simulink model "SunSensor"  (R2025b)
settings: Solver=VariableStepAuto  StartTime=0.0  StopTime=10  RelTol=1e-3
settings Model: Creator=brien  LastModifiedBy=chass

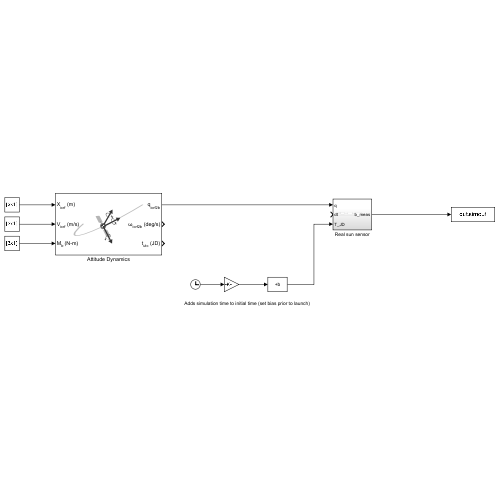
[thumbnail: Simulink's stored preview of the top-level diagram]
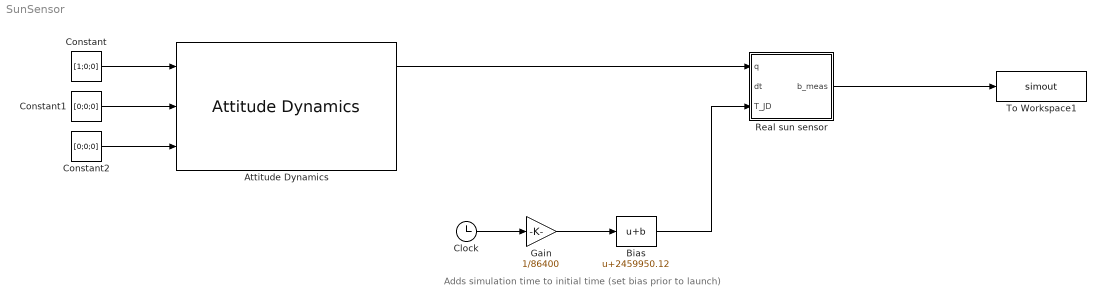
== system SunSensor ==
  note: Adds simulation time to initial time (set bias prior to launch)
  Attitude Dynamics : AttitudeDynamics
  Bias : Bias  Bias=2459950.12  SaturateOnIntegerOverflow=off
  Clock : Clock
  Constant : Constant  Value=[1;0;0]  VectorParams1D=off
  Constant1 : Constant  Value=[0;0;0]  VectorParams1D=off
  Constant2 : Constant  Value=[0;0;0]  VectorParams1D=off
  Gain : Gain  Gain=1/86400
  Real sun sensor : Subsystem
  To Workspace1 : ToWorkspace  VariableName=simout  SampleTime=-1
  wires:
  Constant/1 -> Attitude Dynamics/1
  Constant1/1 -> Attitude Dynamics/2
  Constant2/1 -> Attitude Dynamics/3
  Clock/1 -> Gain/1
  Gain/1 -> Bias/1
  Attitude Dynamics/1 -> Real sun sensor/1(q)
  Bias/1 -> Real sun sensor/3(T_JD)
  Real sun sensor/1(b_meas) -> To Workspace1/1

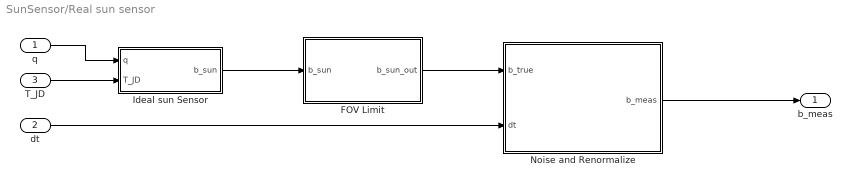
== system SunSensor/Real sun sensor ==
  q : Inport
  dt : Inport  Port=2
  T_JD : Inport  Port=3
  FOV Limit : MATLAB Function  TreatAsAtomicUnit=on
  Ideal sun Sensor : Subsystem
  Noise and Renormalize : MATLAB Function  TreatAsAtomicUnit=on
  b_meas : Outport
  wires:
  dt/1 -> Noise and Renormalize/2(dt)
  Ideal sun Sensor/1(b_sun) -> FOV Limit/1(b_sun)
  FOV Limit/1(b_sun_out) -> Noise and Renormalize/1(b_true)
  Noise and Renormalize/1(b_meas) -> b_meas/1
  T_JD/1 -> Ideal sun Sensor/2(T_JD)
  q/1 -> Ideal sun Sensor/1(q)

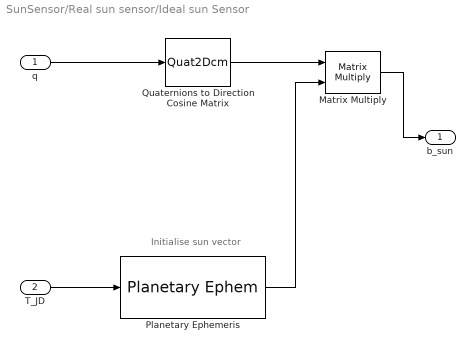
== system SunSensor/Real sun sensor/Ideal sun Sensor ==
  note: Initialise sun vector
  q : Inport
  T_JD : Inport  Port=2
  Matrix Multiply : Product  Multiplication=Matrix(*)
  Planetary Ephemeris : PlanetaryEphem  units=m,m/s  target=Sun  outputVelocity=off
  Quaternions to Direction Cosine Matrix : Quat2Dcm
  b_sun : Outport
  wires:
  q/1 -> Quaternions to Direction Cosine Matrix/1
  Quaternions to Direction Cosine Matrix/1 -> Matrix Multiply/1
  Matrix Multiply/1 -> b_sun/1
  Planetary Ephemeris/1 -> Matrix Multiply/2
  T_JD/1 -> Planetary Ephemeris/1

== matlab function SunSensor/Real sun sensor/Noise and Renormalize ==
  settings: updateMethod=DISCRETE
  data: b_true input; b_meas output; dt input
function b_meas = sunSensorVector(b_true, dt)
% b_true : 3x1 true Sun vector (unit vector) in the body frame of reference ?
% dt     : simulation timestep (s)

% Output:
% b_meas : 3x1 measured Sun vector (unit vector) in the body frame of reference ?
%          with noise, slew-rate limit, and normalized

    sigma_angle = deg2rad(0.1);   % 1-sigma noise (from 0.2° 2-sigma spec)
    slew_max    = deg2rad(70);    % max change per second

    
    % 1) Add Gaussian noise (small vector perturbation)
    
    noise = sigma_angle * randn(3,1);
    b_noisy = b_true(:) + noise;

    
    % 2) Apply slew-rate limit
    
    persistent b_prev;
    if isempty(b_prev)
        b_prev = b_noisy;
    end

    delta = b_noisy - b_prev;
    delta_norm = norm(delta);
    max_step = slew_max * dt;

    if delta_norm > max_step
        delta = delta * (max_step / delta_norm);
    end

    b_slew = b_prev + delta;
    b_prev = b_slew;

    
    % 3) Normalize to unit vector
    
    b_meas = b_slew / norm(b_slew);

end

== matlab function SunSensor/Real sun sensor/FOV Limit ==
  data: b_sun input; b_sun_out output
function b_sun_out = sunSensorFOV(b_sun)
    % Sun Sensor FOV Implementation
    %
    % Input:
    %   b_sun       - 3x1 Sun vector in body frame
    % Output:
    %   b_sun_out   - 3x1 Sun vector with FOV applied

    % --- Parameters ---
    alpha = 180;                 % FOV half-angle in degrees
    sensor_axis = [1; 0; 0];    % Sensor pointing along body x-axis

    % Normalize vectors
    b_sun_norm = b_sun / norm(b_sun);
    sensor_axis_norm = sensor_axis / norm(sensor_axis);

    % Compute angle between Sun vector and sensor axis
    cos_theta = dot(b_sun_norm, sensor_axis_norm);
    theta_deg = acosd(cos_theta);  % angle in degrees

    % Apply FOV
    if theta_deg <= alpha
        b_sun_out = b_sun;      % Sun visible
    else
        b_sun_out = [0; 0; 0];  % Sun outside FOV
    end
end
